simulink model "gm_fourxfour_designfxdpt_givens"  (R2018b)
settings: Solver=FixedStepDiscrete  StartTime=0.0  StopTime=0.18e-6  RelTol=1e-3
InitFcn:
  | if isempty(which('mylib'))
  |      tmp = fileparts(which(bdroot));
  |      run(fullfile(fileparts(tmp), '5-Utilities', 'addPathsPfcHw.m'));
  | end
  | 
  | data_types_givens
StopFcn:
  | GivensSim_Stop
undefined symbols (not defined in the file or in its folder): f
(part 3 of 3)

== system gm_fourxfour_designfxdpt_givens/fourxfour_designfxdpt/Givens_Internal_QR_Cell/Delay ==
  in0 : Inport  OutDataTypeStr=fixdt(1, 24, 14)  SampleTime=1e-08
  Enable_out11 : EnablePort  OutDataTypeStr=boolean
  Delay : Delay  DelayLength=double(1)  InitialCondition=0  InputProcessing=Inherited
  out0 : Outport  OutDataTypeStr=fixdt(1, 24, 14)  InitialOutput=0
  wires:
  Delay/1 -> out0/1
  in0/1 -> Delay/1

== system gm_fourxfour_designfxdpt_givens/fourxfour_designfxdpt/Givens_Internal_QR_Cell/Delay1 ==
  in0 : Inport  OutDataTypeStr=fixdt(1, 24, 14)  SampleTime=1e-08
  Enable_out11 : EnablePort  OutDataTypeStr=boolean
  Delay1 : Delay  DelayLength=double(1)  InitialCondition=0  InputProcessing=Inherited
  out0 : Outport  OutDataTypeStr=fixdt(1, 24, 14)  InitialOutput=0
  wires:
  Delay1/1 -> out0/1
  in0/1 -> Delay1/1

== system gm_fourxfour_designfxdpt_givens/fourxfour_designfxdpt/Givens_Internal_QR_Cell/complex_mul ==
  In1_r : Inport  OutDataTypeStr=fixdt(1, 24, 14)  PortDimensions=1  SampleTime=1e-08
  In1_i : Inport  Port=2  OutDataTypeStr=fixdt(1, 24, 14)  PortDimensions=1  SampleTime=1e-08
  In2_r : Inport  Port=3  OutDataTypeStr=fixdt(1, 24, 14)  PortDimensions=1  SampleTime=1e-08
  In2_i : Inport  Port=4  OutDataTypeStr=fixdt(1, 24, 14)  PortDimensions=1  SampleTime=1e-08
  Add : Sum  Inputs=+-
  Add1 : Sum
  Product{,1..3} (4 alike) : Product
  Out1_r : Outport  InitialOutput=0
  Out1_i : Outport  Port=2  InitialOutput=0
  wires:
  In1_r/1 -> Product3/1, Product/1
  In1_i/1 -> Product2/1, Product1/1
  In2_r/1 -> Product2/2, Product/2
  In2_i/1 -> Product3/2, Product1/2
  Add/1 -> Out1_r/1
  Add1/1 -> Out1_i/1
  Product/1 -> Add/1
  Product1/1 -> Add/2
  Product2/1 -> Add1/1
  Product3/1 -> Add1/2

== system gm_fourxfour_designfxdpt_givens/fourxfour_designfxdpt/Givens_Internal_QR_Cell/complex_mul1 ==
  In1_r : Inport  OutDataTypeStr=fixdt(1, 24, 14)  PortDimensions=1  SampleTime=1e-08
  In1_i : Inport  Port=2  OutDataTypeStr=fixdt(1, 24, 14)  PortDimensions=1  SampleTime=1e-08
  In2_r : Inport  Port=3  OutDataTypeStr=fixdt(1, 24, 14)  PortDimensions=1  SampleTime=1e-08
  In2_i : Inport  Port=4  OutDataTypeStr=fixdt(1, 24, 14)  PortDimensions=1  SampleTime=1e-08
  Add : Sum  Inputs=+-
  Add1 : Sum
  Product{,1..3} (4 alike) : Product
  Out1_r : Outport  InitialOutput=0
  Out1_i : Outport  Port=2  InitialOutput=0
  wires:
  In1_r/1 -> Product3/1, Product/1
  In1_i/1 -> Product2/1, Product1/1
  In2_r/1 -> Product2/2, Product/2
  In2_i/1 -> Product3/2, Product1/2
  Add/1 -> Out1_r/1
  Add1/1 -> Out1_i/1
  Product/1 -> Add/1
  Product1/1 -> Add/2
  Product2/1 -> Add1/1
  Product3/1 -> Add1/2

== system gm_fourxfour_designfxdpt_givens/fourxfour_designfxdpt/Givens_Internal_QR_Cell/complex_mul_rz1 ==
  In1_r : Inport  OutDataTypeStr=fixdt(1, 24, 14)  PortDimensions=1  SampleTime=1e-08
  In1_i : Inport  Port=2  OutDataTypeStr=fixdt(1, 24, 14)  PortDimensions=1  SampleTime=1e-08
  In2_r : Inport  Port=3  OutDataTypeStr=fixdt(1, 24, 14)  PortDimensions=1  SampleTime=1e-08
  In2_i : Inport  Port=4  OutDataTypeStr=fixdt(1, 24, 14)  PortDimensions=1  SampleTime=1e-08
  Add : Sum  Inputs=+-
  Add1 : Sum
  Data Type Conversion{1..3,13} (4 alike) : DataTypeConversion  OutDataTypeStr=data1
  Product{,1..3} (4 alike) : Product
  Out1_r : Outport  InitialOutput=0
  Out1_i : Outport  Port=2  InitialOutput=0
  wires:
  In1_r/1 -> Product3/1, Product/1
  In1_i/1 -> Product2/1, Product1/1
  In2_r/1 -> Product2/2, Product/2
  In2_i/1 -> Product3/2, Product1/2
  Add/1 -> Out1_r/1
  Add1/1 -> Out1_i/1
  Data Type Conversion1/1 -> Add/2
  Data Type Conversion13/1 -> Add/1
  Data Type Conversion2/1 -> Add1/1
  Data Type Conversion3/1 -> Add1/2
  Product/1 -> Data Type Conversion13/1
  Product1/1 -> Data Type Conversion1/1
  Product2/1 -> Data Type Conversion2/1
  Product3/1 -> Data Type Conversion3/1

== system gm_fourxfour_designfxdpt_givens/fourxfour_designfxdpt/Givens_Internal_QR_Cell1/Delay ==
  in0 : Inport  OutDataTypeStr=fixdt(1, 24, 14)  SampleTime=1e-08
  Enable_out11 : EnablePort  OutDataTypeStr=boolean
  Delay : Delay  DelayLength=double(1)  InitialCondition=0  InputProcessing=Inherited
  out0 : Outport  OutDataTypeStr=fixdt(1, 24, 14)  InitialOutput=0
  wires:
  Delay/1 -> out0/1
  in0/1 -> Delay/1

== system gm_fourxfour_designfxdpt_givens/fourxfour_designfxdpt/Givens_Internal_QR_Cell1/Delay1 ==
  in0 : Inport  OutDataTypeStr=fixdt(1, 24, 14)  SampleTime=1e-08
  Enable_out11 : EnablePort  OutDataTypeStr=boolean
  Delay1 : Delay  DelayLength=double(1)  InitialCondition=0  InputProcessing=Inherited
  out0 : Outport  OutDataTypeStr=fixdt(1, 24, 14)  InitialOutput=0
  wires:
  Delay1/1 -> out0/1
  in0/1 -> Delay1/1

== system gm_fourxfour_designfxdpt_givens/fourxfour_designfxdpt/Givens_Internal_QR_Cell1/complex_mul ==
  In1_r : Inport  OutDataTypeStr=fixdt(1, 24, 14)  PortDimensions=1  SampleTime=1e-08
  In1_i : Inport  Port=2  OutDataTypeStr=fixdt(1, 24, 14)  PortDimensions=1  SampleTime=1e-08
  In2_r : Inport  Port=3  OutDataTypeStr=fixdt(1, 24, 14)  PortDimensions=1  SampleTime=1e-08
  In2_i : Inport  Port=4  OutDataTypeStr=fixdt(1, 24, 14)  PortDimensions=1  SampleTime=1e-08
  Add : Sum  Inputs=+-
  Add1 : Sum
  Product{,1..3} (4 alike) : Product
  Out1_r : Outport  InitialOutput=0
  Out1_i : Outport  Port=2  InitialOutput=0
  wires:
  In1_r/1 -> Product3/1, Product/1
  In1_i/1 -> Product2/1, Product1/1
  In2_r/1 -> Product2/2, Product/2
  In2_i/1 -> Product3/2, Product1/2
  Add/1 -> Out1_r/1
  Add1/1 -> Out1_i/1
  Product/1 -> Add/1
  Product1/1 -> Add/2
  Product2/1 -> Add1/1
  Product3/1 -> Add1/2

== system gm_fourxfour_designfxdpt_givens/fourxfour_designfxdpt/Givens_Internal_QR_Cell1/complex_mul1 ==
  In1_r : Inport  OutDataTypeStr=fixdt(1, 24, 14)  PortDimensions=1  SampleTime=1e-08
  In1_i : Inport  Port=2  OutDataTypeStr=fixdt(1, 24, 14)  PortDimensions=1  SampleTime=1e-08
  In2_r : Inport  Port=3  OutDataTypeStr=fixdt(1, 24, 14)  PortDimensions=1  SampleTime=1e-08
  In2_i : Inport  Port=4  OutDataTypeStr=fixdt(1, 24, 14)  PortDimensions=1  SampleTime=1e-08
  Add : Sum  Inputs=+-
  Add1 : Sum
  Product{,1..3} (4 alike) : Product
  Out1_r : Outport  InitialOutput=0
  Out1_i : Outport  Port=2  InitialOutput=0
  wires:
  In1_r/1 -> Product3/1, Product/1
  In1_i/1 -> Product2/1, Product1/1
  In2_r/1 -> Product2/2, Product/2
  In2_i/1 -> Product3/2, Product1/2
  Add/1 -> Out1_r/1
  Add1/1 -> Out1_i/1
  Product/1 -> Add/1
  Product1/1 -> Add/2
  Product2/1 -> Add1/1
  Product3/1 -> Add1/2

== system gm_fourxfour_designfxdpt_givens/fourxfour_designfxdpt/Givens_Internal_QR_Cell1/complex_mul_rz1 ==
  In1_r : Inport  OutDataTypeStr=fixdt(1, 24, 14)  PortDimensions=1  SampleTime=1e-08
  In1_i : Inport  Port=2  OutDataTypeStr=fixdt(1, 24, 14)  PortDimensions=1  SampleTime=1e-08
  In2_r : Inport  Port=3  OutDataTypeStr=fixdt(1, 24, 14)  PortDimensions=1  SampleTime=1e-08
  In2_i : Inport  Port=4  OutDataTypeStr=fixdt(1, 24, 14)  PortDimensions=1  SampleTime=1e-08
  Add : Sum  Inputs=+-
  Add1 : Sum
  Data Type Conversion{1..3,13} (4 alike) : DataTypeConversion  OutDataTypeStr=data1
  Product{,1..3} (4 alike) : Product
  Out1_r : Outport  InitialOutput=0
  Out1_i : Outport  Port=2  InitialOutput=0
  wires:
  In1_r/1 -> Product3/1, Product/1
  In1_i/1 -> Product2/1, Product1/1
  In2_r/1 -> Product2/2, Product/2
  In2_i/1 -> Product3/2, Product1/2
  Add/1 -> Out1_r/1
  Add1/1 -> Out1_i/1
  Data Type Conversion1/1 -> Add/2
  Data Type Conversion13/1 -> Add/1
  Data Type Conversion2/1 -> Add1/1
  Data Type Conversion3/1 -> Add1/2
  Product/1 -> Data Type Conversion13/1
  Product1/1 -> Data Type Conversion1/1
  Product2/1 -> Data Type Conversion2/1
  Product3/1 -> Data Type Conversion3/1

== system gm_fourxfour_designfxdpt_givens/fourxfour_designfxdpt/Givens_Internal_QR_Cell2/Delay ==
  in0 : Inport  OutDataTypeStr=fixdt(1, 24, 14)  SampleTime=1e-08
  Enable_out11 : EnablePort  OutDataTypeStr=boolean
  Delay : Delay  DelayLength=double(1)  InitialCondition=0  InputProcessing=Inherited
  out0 : Outport  OutDataTypeStr=fixdt(1, 24, 14)  InitialOutput=0
  wires:
  Delay/1 -> out0/1
  in0/1 -> Delay/1

== system gm_fourxfour_designfxdpt_givens/fourxfour_designfxdpt/Givens_Internal_QR_Cell2/Delay1 ==
  in0 : Inport  OutDataTypeStr=fixdt(1, 24, 14)  SampleTime=1e-08
  Enable_out11 : EnablePort  OutDataTypeStr=boolean
  Delay1 : Delay  DelayLength=double(1)  InitialCondition=0  InputProcessing=Inherited
  out0 : Outport  OutDataTypeStr=fixdt(1, 24, 14)  InitialOutput=0
  wires:
  Delay1/1 -> out0/1
  in0/1 -> Delay1/1

== system gm_fourxfour_designfxdpt_givens/fourxfour_designfxdpt/Givens_Internal_QR_Cell2/complex_mul ==
  In1_r : Inport  OutDataTypeStr=fixdt(1, 24, 14)  PortDimensions=1  SampleTime=1e-08
  In1_i : Inport  Port=2  OutDataTypeStr=fixdt(1, 24, 14)  PortDimensions=1  SampleTime=1e-08
  In2_r : Inport  Port=3  OutDataTypeStr=fixdt(1, 24, 14)  PortDimensions=1  SampleTime=1e-08
  In2_i : Inport  Port=4  OutDataTypeStr=fixdt(1, 24, 14)  PortDimensions=1  SampleTime=1e-08
  Add : Sum  Inputs=+-
  Add1 : Sum
  Product{,1..3} (4 alike) : Product
  Out1_r : Outport  InitialOutput=0
  Out1_i : Outport  Port=2  InitialOutput=0
  wires:
  In1_r/1 -> Product3/1, Product/1
  In1_i/1 -> Product2/1, Product1/1
  In2_r/1 -> Product2/2, Product/2
  In2_i/1 -> Product3/2, Product1/2
  Add/1 -> Out1_r/1
  Add1/1 -> Out1_i/1
  Product/1 -> Add/1
  Product1/1 -> Add/2
  Product2/1 -> Add1/1
  Product3/1 -> Add1/2

== system gm_fourxfour_designfxdpt_givens/fourxfour_designfxdpt/Givens_Internal_QR_Cell2/complex_mul1 ==
  In1_r : Inport  OutDataTypeStr=fixdt(1, 24, 14)  PortDimensions=1  SampleTime=1e-08
  In1_i : Inport  Port=2  OutDataTypeStr=fixdt(1, 24, 14)  PortDimensions=1  SampleTime=1e-08
  In2_r : Inport  Port=3  OutDataTypeStr=fixdt(1, 24, 14)  PortDimensions=1  SampleTime=1e-08
  In2_i : Inport  Port=4  OutDataTypeStr=fixdt(1, 24, 14)  PortDimensions=1  SampleTime=1e-08
  Add : Sum  Inputs=+-
  Add1 : Sum
  Product{,1..3} (4 alike) : Product
  Out1_r : Outport  InitialOutput=0
  Out1_i : Outport  Port=2  InitialOutput=0
  wires:
  In1_r/1 -> Product3/1, Product/1
  In1_i/1 -> Product2/1, Product1/1
  In2_r/1 -> Product2/2, Product/2
  In2_i/1 -> Product3/2, Product1/2
  Add/1 -> Out1_r/1
  Add1/1 -> Out1_i/1
  Product/1 -> Add/1
  Product1/1 -> Add/2
  Product2/1 -> Add1/1
  Product3/1 -> Add1/2

== system gm_fourxfour_designfxdpt_givens/fourxfour_designfxdpt/Givens_Internal_QR_Cell2/complex_mul_rz1 ==
  In1_r : Inport  OutDataTypeStr=fixdt(1, 24, 14)  PortDimensions=1  SampleTime=1e-08
  In1_i : Inport  Port=2  OutDataTypeStr=fixdt(1, 24, 14)  PortDimensions=1  SampleTime=1e-08
  In2_r : Inport  Port=3  OutDataTypeStr=fixdt(1, 24, 14)  PortDimensions=1  SampleTime=1e-08
  In2_i : Inport  Port=4  OutDataTypeStr=fixdt(1, 24, 14)  PortDimensions=1  SampleTime=1e-08
  Add : Sum  Inputs=+-
  Add1 : Sum
  Data Type Conversion{1..3,13} (4 alike) : DataTypeConversion  OutDataTypeStr=data1
  Product{,1..3} (4 alike) : Product
  Out1_r : Outport  InitialOutput=0
  Out1_i : Outport  Port=2  InitialOutput=0
  wires:
  In1_r/1 -> Product3/1, Product/1
  In1_i/1 -> Product2/1, Product1/1
  In2_r/1 -> Product2/2, Product/2
  In2_i/1 -> Product3/2, Product1/2
  Add/1 -> Out1_r/1
  Add1/1 -> Out1_i/1
  Data Type Conversion1/1 -> Add/2
  Data Type Conversion13/1 -> Add/1
  Data Type Conversion2/1 -> Add1/1
  Data Type Conversion3/1 -> Add1/2
  Product/1 -> Data Type Conversion13/1
  Product1/1 -> Data Type Conversion1/1
  Product2/1 -> Data Type Conversion2/1
  Product3/1 -> Data Type Conversion3/1

== system gm_fourxfour_designfxdpt_givens/fourxfour_designfxdpt/Givens_Internal_QR_Cell3/Delay ==
  in0 : Inport  OutDataTypeStr=fixdt(1, 24, 14)  SampleTime=1e-08
  Enable_out11 : EnablePort  OutDataTypeStr=boolean
  Delay : Delay  DelayLength=double(1)  InitialCondition=0  InputProcessing=Inherited
  out0 : Outport  OutDataTypeStr=fixdt(1, 24, 14)  InitialOutput=0
  wires:
  Delay/1 -> out0/1
  in0/1 -> Delay/1

== system gm_fourxfour_designfxdpt_givens/fourxfour_designfxdpt/Givens_Internal_QR_Cell3/Delay1 ==
  in0 : Inport  OutDataTypeStr=fixdt(1, 24, 14)  SampleTime=1e-08
  Enable_out11 : EnablePort  OutDataTypeStr=boolean
  Delay1 : Delay  DelayLength=double(1)  InitialCondition=0  InputProcessing=Inherited
  out0 : Outport  OutDataTypeStr=fixdt(1, 24, 14)  InitialOutput=0
  wires:
  Delay1/1 -> out0/1
  in0/1 -> Delay1/1

== system gm_fourxfour_designfxdpt_givens/fourxfour_designfxdpt/Givens_Internal_QR_Cell3/complex_mul ==
  In1_r : Inport  OutDataTypeStr=fixdt(1, 24, 14)  PortDimensions=1  SampleTime=1e-08
  In1_i : Inport  Port=2  OutDataTypeStr=fixdt(1, 24, 14)  PortDimensions=1  SampleTime=1e-08
  In2_r : Inport  Port=3  OutDataTypeStr=fixdt(1, 24, 14)  PortDimensions=1  SampleTime=1e-08
  In2_i : Inport  Port=4  OutDataTypeStr=fixdt(1, 24, 14)  PortDimensions=1  SampleTime=1e-08
  Add : Sum  Inputs=+-
  Add1 : Sum
  Product{,1..3} (4 alike) : Product
  Out1_r : Outport  InitialOutput=0
  Out1_i : Outport  Port=2  InitialOutput=0
  wires:
  In1_r/1 -> Product3/1, Product/1
  In1_i/1 -> Product2/1, Product1/1
  In2_r/1 -> Product2/2, Product/2
  In2_i/1 -> Product3/2, Product1/2
  Add/1 -> Out1_r/1
  Add1/1 -> Out1_i/1
  Product/1 -> Add/1
  Product1/1 -> Add/2
  Product2/1 -> Add1/1
  Product3/1 -> Add1/2

== system gm_fourxfour_designfxdpt_givens/fourxfour_designfxdpt/Givens_Internal_QR_Cell3/complex_mul1 ==
  In1_r : Inport  OutDataTypeStr=fixdt(1, 24, 14)  PortDimensions=1  SampleTime=1e-08
  In1_i : Inport  Port=2  OutDataTypeStr=fixdt(1, 24, 14)  PortDimensions=1  SampleTime=1e-08
  In2_r : Inport  Port=3  OutDataTypeStr=fixdt(1, 24, 14)  PortDimensions=1  SampleTime=1e-08
  In2_i : Inport  Port=4  OutDataTypeStr=fixdt(1, 24, 14)  PortDimensions=1  SampleTime=1e-08
  Add : Sum  Inputs=+-
  Add1 : Sum
  Product{,1..3} (4 alike) : Product
  Out1_r : Outport  InitialOutput=0
  Out1_i : Outport  Port=2  InitialOutput=0
  wires:
  In1_r/1 -> Product3/1, Product/1
  In1_i/1 -> Product2/1, Product1/1
  In2_r/1 -> Product2/2, Product/2
  In2_i/1 -> Product3/2, Product1/2
  Add/1 -> Out1_r/1
  Add1/1 -> Out1_i/1
  Product/1 -> Add/1
  Product1/1 -> Add/2
  Product2/1 -> Add1/1
  Product3/1 -> Add1/2

== system gm_fourxfour_designfxdpt_givens/fourxfour_designfxdpt/Givens_Internal_QR_Cell3/complex_mul_rz1 ==
  In1_r : Inport  OutDataTypeStr=fixdt(1, 24, 14)  PortDimensions=1  SampleTime=1e-08
  In1_i : Inport  Port=2  OutDataTypeStr=fixdt(1, 24, 14)  PortDimensions=1  SampleTime=1e-08
  In2_r : Inport  Port=3  OutDataTypeStr=fixdt(1, 24, 14)  PortDimensions=1  SampleTime=1e-08
  In2_i : Inport  Port=4  OutDataTypeStr=fixdt(1, 24, 14)  PortDimensions=1  SampleTime=1e-08
  Add : Sum  Inputs=+-
  Add1 : Sum
  Data Type Conversion{1..3,13} (4 alike) : DataTypeConversion  OutDataTypeStr=data1
  Product{,1..3} (4 alike) : Product
  Out1_r : Outport  InitialOutput=0
  Out1_i : Outport  Port=2  InitialOutput=0
  wires:
  In1_r/1 -> Product3/1, Product/1
  In1_i/1 -> Product2/1, Product1/1
  In2_r/1 -> Product2/2, Product/2
  In2_i/1 -> Product3/2, Product1/2
  Add/1 -> Out1_r/1
  Add1/1 -> Out1_i/1
  Data Type Conversion1/1 -> Add/2
  Data Type Conversion13/1 -> Add/1
  Data Type Conversion2/1 -> Add1/1
  Data Type Conversion3/1 -> Add1/2
  Product/1 -> Data Type Conversion13/1
  Product1/1 -> Data Type Conversion1/1
  Product2/1 -> Data Type Conversion2/1
  Product3/1 -> Data Type Conversion3/1

== system gm_fourxfour_designfxdpt_givens/fourxfour_designfxdpt/Givens_Internal_QR_Cell4/Delay ==
  in0 : Inport  OutDataTypeStr=fixdt(1, 24, 14)  SampleTime=1e-08
  Enable_out11 : EnablePort  OutDataTypeStr=boolean
  Delay : Delay  DelayLength=double(1)  InitialCondition=0  InputProcessing=Inherited
  out0 : Outport  OutDataTypeStr=fixdt(1, 24, 14)  InitialOutput=0
  wires:
  Delay/1 -> out0/1
  in0/1 -> Delay/1

== system gm_fourxfour_designfxdpt_givens/fourxfour_designfxdpt/Givens_Internal_QR_Cell4/Delay1 ==
  in0 : Inport  OutDataTypeStr=fixdt(1, 24, 14)  SampleTime=1e-08
  Enable_out11 : EnablePort  OutDataTypeStr=boolean
  Delay1 : Delay  DelayLength=double(1)  InitialCondition=0  InputProcessing=Inherited
  out0 : Outport  OutDataTypeStr=fixdt(1, 24, 14)  InitialOutput=0
  wires:
  Delay1/1 -> out0/1
  in0/1 -> Delay1/1

== system gm_fourxfour_designfxdpt_givens/fourxfour_designfxdpt/Givens_Internal_QR_Cell4/complex_mul ==
  In1_r : Inport  OutDataTypeStr=fixdt(1, 24, 14)  PortDimensions=1  SampleTime=1e-08
  In1_i : Inport  Port=2  OutDataTypeStr=fixdt(1, 24, 14)  PortDimensions=1  SampleTime=1e-08
  In2_r : Inport  Port=3  OutDataTypeStr=fixdt(1, 24, 14)  PortDimensions=1  SampleTime=1e-08
  In2_i : Inport  Port=4  OutDataTypeStr=fixdt(1, 24, 14)  PortDimensions=1  SampleTime=1e-08
  Add : Sum  Inputs=+-
  Add1 : Sum
  Product{,1..3} (4 alike) : Product
  Out1_r : Outport  InitialOutput=0
  Out1_i : Outport  Port=2  InitialOutput=0
  wires:
  In1_r/1 -> Product3/1, Product/1
  In1_i/1 -> Product2/1, Product1/1
  In2_r/1 -> Product2/2, Product/2
  In2_i/1 -> Product3/2, Product1/2
  Add/1 -> Out1_r/1
  Add1/1 -> Out1_i/1
  Product/1 -> Add/1
  Product1/1 -> Add/2
  Product2/1 -> Add1/1
  Product3/1 -> Add1/2

== system gm_fourxfour_designfxdpt_givens/fourxfour_designfxdpt/Givens_Internal_QR_Cell4/complex_mul1 ==
  In1_r : Inport  OutDataTypeStr=fixdt(1, 24, 14)  PortDimensions=1  SampleTime=1e-08
  In1_i : Inport  Port=2  OutDataTypeStr=fixdt(1, 24, 14)  PortDimensions=1  SampleTime=1e-08
  In2_r : Inport  Port=3  OutDataTypeStr=fixdt(1, 24, 14)  PortDimensions=1  SampleTime=1e-08
  In2_i : Inport  Port=4  OutDataTypeStr=fixdt(1, 24, 14)  PortDimensions=1  SampleTime=1e-08
  Add : Sum  Inputs=+-
  Add1 : Sum
  Product{,1..3} (4 alike) : Product
  Out1_r : Outport  InitialOutput=0
  Out1_i : Outport  Port=2  InitialOutput=0
  wires:
  In1_r/1 -> Product3/1, Product/1
  In1_i/1 -> Product2/1, Product1/1
  In2_r/1 -> Product2/2, Product/2
  In2_i/1 -> Product3/2, Product1/2
  Add/1 -> Out1_r/1
  Add1/1 -> Out1_i/1
  Product/1 -> Add/1
  Product1/1 -> Add/2
  Product2/1 -> Add1/1
  Product3/1 -> Add1/2

== system gm_fourxfour_designfxdpt_givens/fourxfour_designfxdpt/Givens_Internal_QR_Cell4/complex_mul_rz1 ==
  In1_r : Inport  OutDataTypeStr=fixdt(1, 24, 14)  PortDimensions=1  SampleTime=1e-08
  In1_i : Inport  Port=2  OutDataTypeStr=fixdt(1, 24, 14)  PortDimensions=1  SampleTime=1e-08
  In2_r : Inport  Port=3  OutDataTypeStr=fixdt(1, 24, 14)  PortDimensions=1  SampleTime=1e-08
  In2_i : Inport  Port=4  OutDataTypeStr=fixdt(1, 24, 14)  PortDimensions=1  SampleTime=1e-08
  Add : Sum  Inputs=+-
  Add1 : Sum
  Data Type Conversion{1..3,13} (4 alike) : DataTypeConversion  OutDataTypeStr=data1
  Product{,1..3} (4 alike) : Product
  Out1_r : Outport  InitialOutput=0
  Out1_i : Outport  Port=2  InitialOutput=0
  wires:
  In1_r/1 -> Product3/1, Product/1
  In1_i/1 -> Product2/1, Product1/1
  In2_r/1 -> Product2/2, Product/2
  In2_i/1 -> Product3/2, Product1/2
  Add/1 -> Out1_r/1
  Add1/1 -> Out1_i/1
  Data Type Conversion1/1 -> Add/2
  Data Type Conversion13/1 -> Add/1
  Data Type Conversion2/1 -> Add1/1
  Data Type Conversion3/1 -> Add1/2
  Product/1 -> Data Type Conversion13/1
  Product1/1 -> Data Type Conversion1/1
  Product2/1 -> Data Type Conversion2/1
  Product3/1 -> Data Type Conversion3/1

== system gm_fourxfour_designfxdpt_givens/fourxfour_designfxdpt/Givens_Internal_QR_Cell5/Delay ==
  in0 : Inport  OutDataTypeStr=fixdt(1, 24, 14)  SampleTime=1e-08
  Enable_out11 : EnablePort  OutDataTypeStr=boolean
  Delay : Delay  DelayLength=double(1)  InitialCondition=0  InputProcessing=Inherited
  out0 : Outport  OutDataTypeStr=fixdt(1, 24, 14)  InitialOutput=0
  wires:
  Delay/1 -> out0/1
  in0/1 -> Delay/1

== system gm_fourxfour_designfxdpt_givens/fourxfour_designfxdpt/Givens_Internal_QR_Cell5/Delay1 ==
  in0 : Inport  OutDataTypeStr=fixdt(1, 24, 14)  SampleTime=1e-08
  Enable_out11 : EnablePort  OutDataTypeStr=boolean
  Delay1 : Delay  DelayLength=double(1)  InitialCondition=0  InputProcessing=Inherited
  out0 : Outport  OutDataTypeStr=fixdt(1, 24, 14)  InitialOutput=0
  wires:
  Delay1/1 -> out0/1
  in0/1 -> Delay1/1

== system gm_fourxfour_designfxdpt_givens/fourxfour_designfxdpt/Givens_Internal_QR_Cell5/complex_mul ==
  In1_r : Inport  OutDataTypeStr=fixdt(1, 24, 14)  PortDimensions=1  SampleTime=1e-08
  In1_i : Inport  Port=2  OutDataTypeStr=fixdt(1, 24, 14)  PortDimensions=1  SampleTime=1e-08
  In2_r : Inport  Port=3  OutDataTypeStr=fixdt(1, 24, 14)  PortDimensions=1  SampleTime=1e-08
  In2_i : Inport  Port=4  OutDataTypeStr=fixdt(1, 24, 14)  PortDimensions=1  SampleTime=1e-08
  Add : Sum  Inputs=+-
  Add1 : Sum
  Product{,1..3} (4 alike) : Product
  Out1_r : Outport  InitialOutput=0
  Out1_i : Outport  Port=2  InitialOutput=0
  wires:
  In1_r/1 -> Product3/1, Product/1
  In1_i/1 -> Product2/1, Product1/1
  In2_r/1 -> Product2/2, Product/2
  In2_i/1 -> Product3/2, Product1/2
  Add/1 -> Out1_r/1
  Add1/1 -> Out1_i/1
  Product/1 -> Add/1
  Product1/1 -> Add/2
  Product2/1 -> Add1/1
  Product3/1 -> Add1/2

== system gm_fourxfour_designfxdpt_givens/fourxfour_designfxdpt/Givens_Internal_QR_Cell5/complex_mul1 ==
  In1_r : Inport  OutDataTypeStr=fixdt(1, 24, 14)  PortDimensions=1  SampleTime=1e-08
  In1_i : Inport  Port=2  OutDataTypeStr=fixdt(1, 24, 14)  PortDimensions=1  SampleTime=1e-08
  In2_r : Inport  Port=3  OutDataTypeStr=fixdt(1, 24, 14)  PortDimensions=1  SampleTime=1e-08
  In2_i : Inport  Port=4  OutDataTypeStr=fixdt(1, 24, 14)  PortDimensions=1  SampleTime=1e-08
  Add : Sum  Inputs=+-
  Add1 : Sum
  Product{,1..3} (4 alike) : Product
  Out1_r : Outport  InitialOutput=0
  Out1_i : Outport  Port=2  InitialOutput=0
  wires:
  In1_r/1 -> Product3/1, Product/1
  In1_i/1 -> Product2/1, Product1/1
  In2_r/1 -> Product2/2, Product/2
  In2_i/1 -> Product3/2, Product1/2
  Add/1 -> Out1_r/1
  Add1/1 -> Out1_i/1
  Product/1 -> Add/1
  Product1/1 -> Add/2
  Product2/1 -> Add1/1
  Product3/1 -> Add1/2

== system gm_fourxfour_designfxdpt_givens/fourxfour_designfxdpt/Givens_Internal_QR_Cell5/complex_mul_rz1 ==
  In1_r : Inport  OutDataTypeStr=fixdt(1, 24, 14)  PortDimensions=1  SampleTime=1e-08
  In1_i : Inport  Port=2  OutDataTypeStr=fixdt(1, 24, 14)  PortDimensions=1  SampleTime=1e-08
  In2_r : Inport  Port=3  OutDataTypeStr=fixdt(1, 24, 14)  PortDimensions=1  SampleTime=1e-08
  In2_i : Inport  Port=4  OutDataTypeStr=fixdt(1, 24, 14)  PortDimensions=1  SampleTime=1e-08
  Add : Sum  Inputs=+-
  Add1 : Sum
  Data Type Conversion{1..3,13} (4 alike) : DataTypeConversion  OutDataTypeStr=data1
  Product{,1..3} (4 alike) : Product
  Out1_r : Outport  InitialOutput=0
  Out1_i : Outport  Port=2  InitialOutput=0
  wires:
  In1_r/1 -> Product3/1, Product/1
  In1_i/1 -> Product2/1, Product1/1
  In2_r/1 -> Product2/2, Product/2
  In2_i/1 -> Product3/2, Product1/2
  Add/1 -> Out1_r/1
  Add1/1 -> Out1_i/1
  Data Type Conversion1/1 -> Add/2
  Data Type Conversion13/1 -> Add/1
  Data Type Conversion2/1 -> Add1/1
  Data Type Conversion3/1 -> Add1/2
  Product/1 -> Data Type Conversion13/1
  Product1/1 -> Data Type Conversion1/1
  Product2/1 -> Data Type Conversion2/1
  Product3/1 -> Data Type Conversion3/1
